simulink model "Impedance_model"  (Simulink 6.4)
settings: Solver=ode15s  SolverMode=SingleTasking  StartTime=0.0  StopTime=3  FixedStep=0.0001  RelTol=1e-9
values from neighbouring files (symbols this model uses):
  dQ = IN(19:21)    [Dynamics.m]    (also in controller.m; direct_kinematics.m = [ dq11; init.m = [ 0.0)
  Q = IN(16:18)    [Dynamics.m]    (also in controller.m; init.m = [ q11)
libraries: simulink_extras x1
settings Model: LastModifiedBy=Administrator
settings SolverCC: MaxConsecutiveMinStep=2
settings DataIOCC: SignalLoggingName=sigsOut
settings DebuggingCC: SolverPrmCheckMsg=none  StrictBusMsg=None
settings HardwareCC: TargetUnknown=on

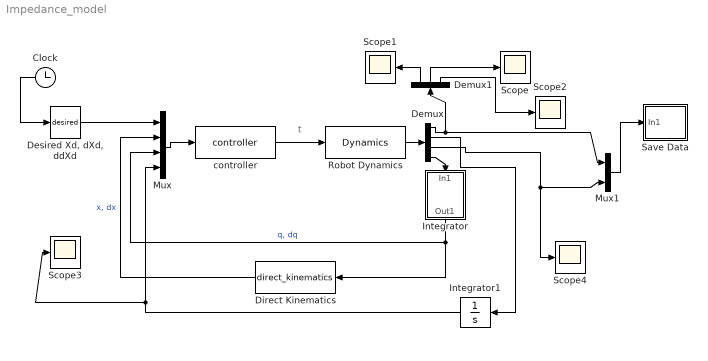
== system Impedance_model ==
  note: t
  Clock : Clock
      settings: Decimation=10
  Demux : Demux  Outputs=[12 1 3 3]
  Demux1 : Demux  Orientation=up  Outputs=[6 3 3]
  "Desired Xd, dXd, ddXd" : MATLABFcn  MATLABFcn=desired
  Direct Kinematics : MATLABFcn  Orientation=left  MATLABFcn=direct_kinematics  OutputDimensions=6
  Integrator : Subsystem  Orientation=down
  Integrator1 : Integrator  Orientation=left
  Mux : Mux  Inputs=[9 6 6 1]
  Mux1 : Mux  Inputs=[12 3]
  Robot Dynamics : MATLABFcn  MATLABFcn=Dynamics  OutputDimensions=19
  Save Data : Subsystem
  Scope{,1..4} (5 alike) : Scope
      Scope settings: YMin=-3.5  YMax=4  SaveName=ScopeData2
      Scope1 settings: YMin=-1.5  YMax=2  SaveName=ScopeData3
      Scope2 settings: YMin=-250  YMax=2500  SaveName=ScopeData4
      Scope3 settings: SaveName=ScopeData5
      Scope4 settings: YMin=-25  YMax=225  SaveName=ScopeData6
  controller : MATLABFcn  MATLABFcn=controller  OutputDimensions=22
  wires:
  Direct Kinematics/1 -> Mux/2  "x, dx"
  controller/1 -> Robot Dynamics/1
  Mux/1 -> controller/1
  Integrator/1(Out1) -> Direct Kinematics/1, Mux/3  "q, dq"
  Robot Dynamics/1 -> Demux/1
  Demux/1 -> Demux1/1, Mux1/1
  Demux1/1 -> Scope1/1
  Demux1/2 -> Scope/1
  Clock/1 -> "Desired Xd, dXd, ddXd"/1
  "Desired Xd, dXd, ddXd"/1 -> Mux/1
  Demux1/3 -> Scope2/1
  Demux/2 -> Integrator1/1
  Integrator1/1 -> Mux/4, Scope3/1
  Demux/4 -> Integrator/1(In1)
  Demux/3 -> Scope4/1, Mux1/2
  Mux1/1 -> Save Data/1(In1)

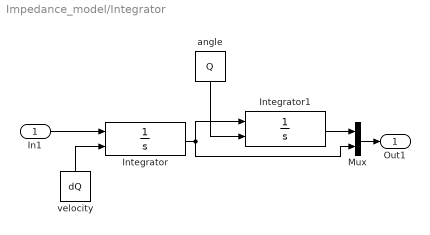
== system Impedance_model/Integrator ==
  In1 : Inport
  Integrator : Integrator  InitialConditionSource=external
  Integrator1 : Integrator  InitialConditionSource=external
  Mux : Mux  Inputs=[3 3]
  angle : Constant  Orientation=down  Value=Q  OutDataType=sfix(16)  ConRadixGroup=Use specified scaling  OutScaling=2^0  SampleTime=inf  FramePeriod=inf
  velocity : Constant  Orientation=up  Value=dQ  OutDataType=sfix(16)  ConRadixGroup=Use specified scaling  OutScaling=2^0  SampleTime=inf  FramePeriod=inf
  Out1 : Outport
  wires:
  Integrator/1 -> Integrator1/1, Mux/2
  velocity/1 -> Integrator/2
  Mux/1 -> Out1/1
  In1/1 -> Integrator/1
  Integrator1/1 -> Mux/1
  angle/1 -> Integrator1/2

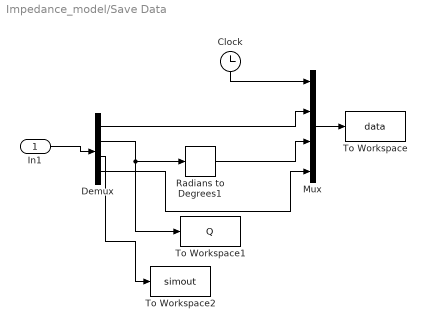
== system Impedance_model/Save Data ==
  In1 : Inport
  Clock : Clock
      settings: Orientation=down  Decimation=10
  Demux : Demux  Outputs=[6 3 3 3]
  Mux : Mux  Inputs=[1 6 3 3]
  Radians to Degrees1 : simulink_extras/Transformations/Radians to Degrees  SystemSampleTime=-1
  To Workspace : ToWorkspace  VariableName=data  SampleTime=0.02  SaveFormat=Array
  To Workspace1 : ToWorkspace  VariableName=Q  SampleTime=0.02  SaveFormat=Array
  To Workspace2 : ToWorkspace  VariableName=simout  SampleTime=-1  SaveFormat=Structure
  wires:
  Mux/1 -> To Workspace/1
  In1/1 -> Demux/1
  Clock/1 -> Mux/1
  Demux/1 -> Mux/2
  Radians to Degrees1/1 -> Mux/3
  Demux/2 -> Radians to Degrees1/1, To Workspace1/1
  Demux/3 -> To Workspace2/1
  Demux/4 -> Mux/4
